simulink library "INT_CoVeh_SpdCoord"  (R2016b)
settings: Solver=VariableStepAuto  StartTime=0.0  StopTime=10.0  RelTol=1e-3
settings Model: Creator=Administrator  LastModifiedBy=Administrator

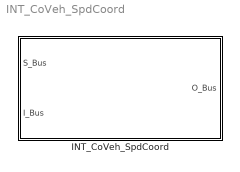
== system INT_CoVeh_SpdCoord ==
  INT_CoVeh_SpdCoord : Subsystem

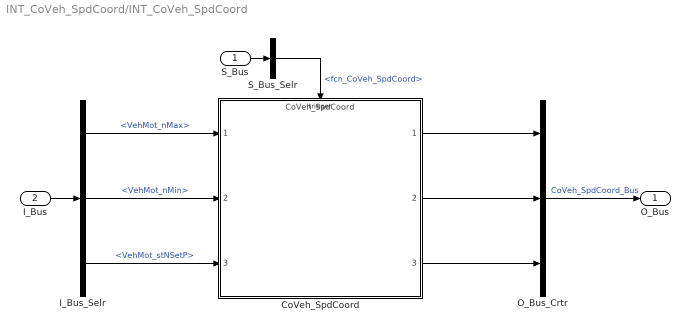
== system INT_CoVeh_SpdCoord/INT_CoVeh_SpdCoord ==
  S_Bus : Inport
  I_Bus : Inport  Port=2
  CoVeh_SpdCoord : ModelReference  ModelNameDialog=CoVeh_SpdCoord  SimulationMode=Normal  ModelReferenceVersion=1.6  TriggerPortName=function  TriggerPortTriggerType=function-call  TriggerPortStatesWhenEnabling=held
  I_Bus_Selr : BusSelector  OutputSignals=VehMot_nMax,VehMot_nMin,VehMot_stNSetP
  O_Bus_Crtr : BusCreator  Inputs=3
  S_Bus_Selr : BusSelector  OutputSignals=fcn_CoVeh_SpdCoord
  O_Bus : Outport
  wires:
  S_Bus_Selr/1 -> CoVeh_SpdCoord/Trigger  "<fcn_CoVeh_SpdCoord>"
  S_Bus/1 -> S_Bus_Selr/1
  I_Bus/1 -> I_Bus_Selr/1
  I_Bus_Selr/1 -> CoVeh_SpdCoord/1  "<VehMot_nMax>"
  I_Bus_Selr/2 -> CoVeh_SpdCoord/2  "<VehMot_nMin>"
  I_Bus_Selr/3 -> CoVeh_SpdCoord/3  "<VehMot_stNSetP>"
  O_Bus_Crtr/1 -> O_Bus/1  "CoVeh_SpdCoord_Bus"
  CoVeh_SpdCoord/1 -> O_Bus_Crtr/1
  CoVeh_SpdCoord/2 -> O_Bus_Crtr/2
  CoVeh_SpdCoord/3 -> O_Bus_Crtr/3
